simulink model "AutoLayoutDemo"  (Simulink 7.8)
settings: Solver=ode45  StartTime=0.0  StopTime=10.0  RelTol=1e-3
settings Model: Creator=postma  LastModifiedBy=monika

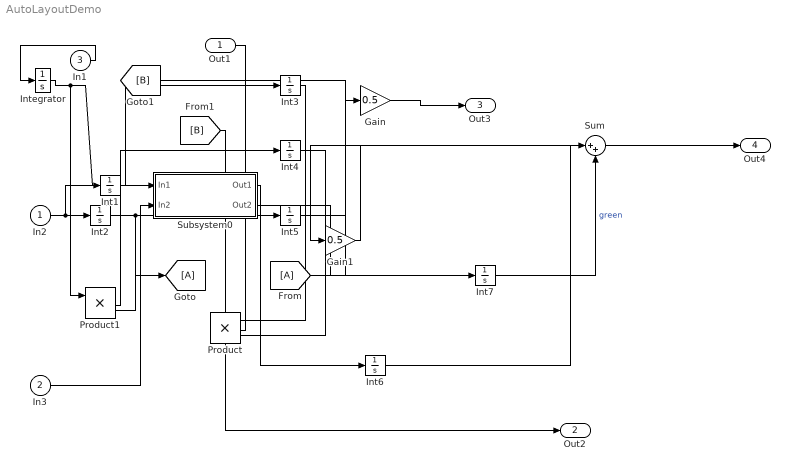
== system AutoLayoutDemo ==
  In2 : Inport
  In3 : Inport  Port=2
  In1 : Inport  Port=3
  Gain : Gain  Gain=0.5
  Gain1 : Gain  Gain=0.5
  Int{1..7} (7 alike) : Integrator
  Integrator : Integrator
  Product : Product  RndMeth=Zero
  Product1 : Product  RndMeth=Zero
  Subsystem0 : Subsystem
  Sum : Sum  Inputs=|++
  Out1 : Outport
  Out2 : Outport  Port=2
  Out3 : Outport  Port=3
  Out4 : Outport  Port=4
  wires:
  Int1/1 -> Int3/1
  Int3/1 -> Product/1
  Product/1 -> Out1/1
  Int4/1 -> Product/2
  Product1/1 -> Int4/1
  Int2/1 -> Product1/2, [A], Int5/1
  In2/1 -> Int2/1, Subsystem0/1(In1)
  In3/1 -> Subsystem0/2(In2)
  Subsystem0/1(Out1) -> Int6/1
  Subsystem0/2(Out2) -> Int7/1
  Gain/1 -> Out3/1
  [A] -> Gain/1
  Sum/1 -> Gain1/1
  Gain1/1 -> Out4/1
  [B] -> Out2/1
  Int5/1 -> [B]
  Int7/1 -> Sum/2  "green"
  Int6/1 -> Sum/1
  Integrator/1 -> Int1/1, Product1/1
  In1/1 -> Integrator/1

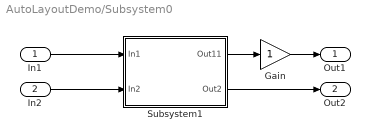
== system AutoLayoutDemo/Subsystem0 ==
  In1 : Inport
  In2 : Inport  Port=2
  Gain : Gain
  Subsystem1 : Subsystem
  Out1 : Outport
  Out2 : Outport  Port=2
  wires:
  In1/1 -> Subsystem1/1(In1)
  Subsystem1/1(Out11) -> Gain/1
  In2/1 -> Subsystem1/2(In2)
  Subsystem1/2(Out2) -> Out2/1
  Gain/1 -> Out1/1

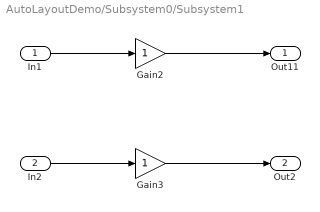
== system AutoLayoutDemo/Subsystem0/Subsystem1 ==
  In1 : Inport
  In2 : Inport  Port=2
  Gain2 : Gain
  Gain3 : Gain
  Out11 : Outport
  Out2 : Outport  Port=2
  wires:
  In1/1 -> Gain2/1
  In2/1 -> Gain3/1
  Gain2/1 -> Out11/1
  Gain3/1 -> Out2/1
